simulink model "Problem_2"  (R2020b)
settings: Solver=VariableStepAuto  StartTime=0.0  StopTime=10.0  MaxStep=0.01  RelTol=1e-3
model workspace (MAT data in the model file):
  B = Simulink.Parameter
  B.Value = 1120
  B.DataType = 'auto'
  B.Dimensions = [1 1]
  k1 = Simulink.Parameter
  k1.Value = 150000
  k1.DataType = 'auto'
  k1.Dimensions = [1 1]
  k2 = Simulink.Parameter
  k2.Value = 310000
  k2.DataType = 'auto'
  k2.Dimensions = [1 1]
  m1 = Simulink.Parameter
  m1.Value = 250
  m1.DataType = 'auto'
  m1.Dimensions = [1 1]
  m2 = Simulink.Parameter
  m2.Value = 50
  m2.DataType = 'auto'
  m2.Dimensions = [1 1]
settings Model: Creator=hp  LastModifiedBy=hp

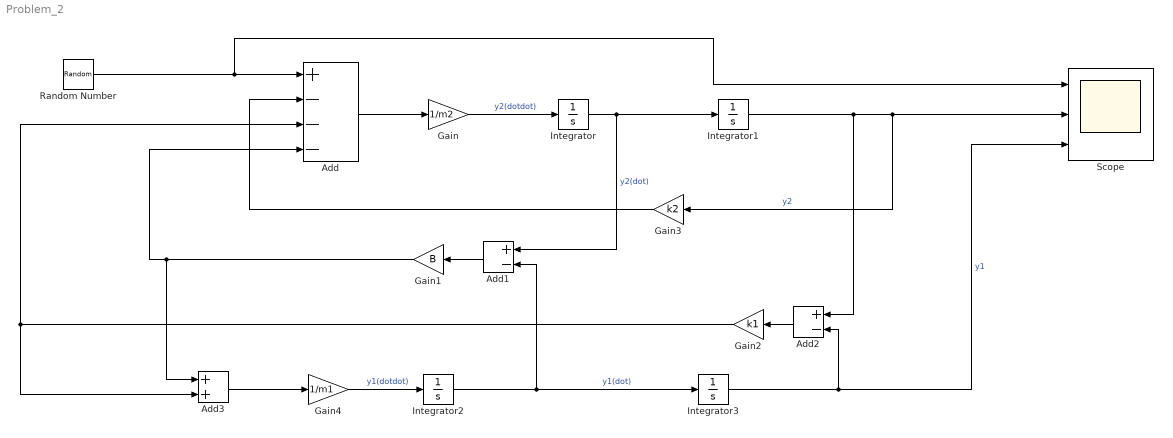
== system Problem_2 ==
  Add : Sum  Inputs=+---
  Add1 : Sum  Inputs=+-
  Add2 : Sum  Inputs=+-
  Add3 : Sum
  Gain : Gain  Gain=1/m2
  Gain1 : Gain  Gain=B
  Gain2 : Gain  Gain=k1
  Gain3 : Gain  Gain=k2
  Gain4 : Gain  Gain=1/m1
  Integrator{,1..3} (4 alike) : Integrator
  Random Number : RandomNumber  SampleTime=0.1
  Scope : Scope  NumInputPorts=3
  wires:
  Random Number/1 -> Add/1, Scope/1
  Add/1 -> Gain/1
  Gain/1 -> Integrator/1  "y2(dotdot)"
  Integrator/1 -> Add1/1, Integrator1/1  "y2(dot)"
  Integrator1/1 -> Add2/1, Gain3/1, Scope/2  "y2"
  Gain1/1 -> Add3/1, Add/4
  Add1/1 -> Gain1/1
  Gain2/1 -> Add3/2, Add/3
  Add2/1 -> Gain2/1
  Gain3/1 -> Add/2
  Gain4/1 -> Integrator2/1  "y1(dotdot)"
  Integrator2/1 -> Add1/2, Integrator3/1  "y1(dot)"
  Integrator3/1 -> Add2/2, Scope/3  "y1"
  Add3/1 -> Gain4/1
